simulink model "x2025_bolier_grupa_07"  (R2023b)
settings: Solver=VariableStepAuto  StartTime=0.0  StopTime=7000  RelTol=1e-3
model workspace (MAT data in the model file):
  Cd = 180
  Csh = 30
  K = 3.1616
  Tauf = 5
  Tf = 8
  Tfuel = 8
  Tw = 6
  k = 3.1616
values from neighbouring files (symbols this model uses):
  A1 = [-1/Tf 0 0 0 ... (first row only)    [Linearyzacja.m]
  A_prim = expm(A1*Ti)    [Dyskretyzacja.m]
  B1 = [1/Tf 0 ... (first row only)    [Linearyzacja.m]
  B_prim = integ*B1    [Dyskretyzacja.m]
  C1 = [0 0 CV 0 ... (first row only)    [Linearyzacja.m]
  CV = 0.5    [Linearyzacja.m]
  CV_FINAL_VALUE = 0.50    (= 0.5)    [INPUT.m]
  CV_INIT_VALUE = 0.5    [INPUT.m]
  D1 = [0 Pt_const ... (first row only)    [Linearyzacja.m]
  Pd_const = 1.025    [Linearyzacja.m]
  SIG = 0.5    [Linearyzacja.m]
  SIG_FINAL_VALUE = 0.3    [INPUT.m]
  SIG_INIT_VALUE = 0.5    [INPUT.m]
  STEP_TIME = 4000    [INPUT.m]
  Ti = 50.0    (= 50)    [Dyskretyzacja.m]
settings Model: Creator=jakub  LastModifiedBy=Filip

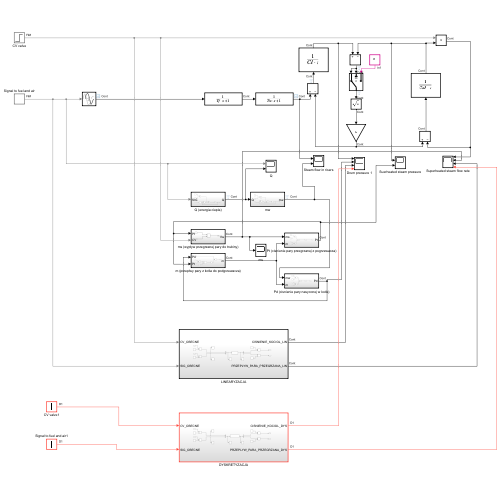
[thumbnail: Simulink's stored preview of the top-level diagram]
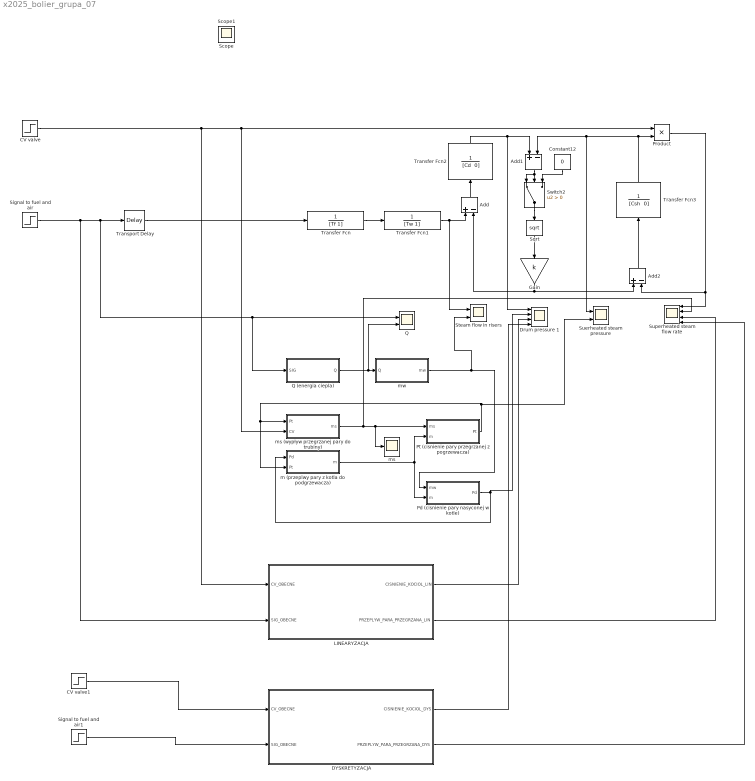
== system x2025_bolier_grupa_07 ==
  " mw " : Subsystem
  Add : Sum  Inputs=+-
  Add1 : Sum  Inputs=+-
  Add2 : Sum  Inputs=+-
  CV valve : Step  Time=STEP_TIME  Before=CV_INIT_VALUE  After=CV_FINAL_VALUE  SampleTime=0
  CV valve1 : Step  Time=STEP_TIME  Before=CV_INIT_VALUE  After=CV_FINAL_VALUE  SampleTime=Ti
  Constant12 : Constant  Value=0
  DYSKRETYZACJA : Subsystem
  Drum pressure 1 : Scope  NumInputPorts=4
  Gain : Gain  Gain=k
  LINEARYZACJA : Subsystem
  Pd (cisnienie pary nasyconej w kotle) : Subsystem
  Product : Product
  Pt (cisnienie pary przegrzanej z pogrzewacza) : Subsystem
  Q : Scope  NumInputPorts=2
  Q (energia ciepla) : Subsystem
  Signal to fuel and air : Step  Time=STEP_TIME  Before=SIG_INIT_VALUE  After=SIG_FINAL_VALUE  SampleTime=0
  Signal to fuel and air1 : Step  Time=STEP_TIME  Before=SIG_INIT_VALUE  After=SIG_FINAL_VALUE  SampleTime=Ti
  Sqrt : Sqrt
  Steam flow in risers : Scope  NumInputPorts=2
  Suerheated steam pressure : Scope  NumInputPorts=2
  Superheated steam flow rate : Scope  NumInputPorts=4
  Switch2 : Switch  Criteria=u2 > Threshold  SaturateOnIntegerOverflow=off  InputSameDT=off
  Transfer Fcn : TransferFcn  Denominator=[Tf 1]
  Transfer Fcn1 : TransferFcn  Denominator=[Tw 1]
  Transfer Fcn2 : TransferFcn  Denominator="[Cd  0]"
  Transfer Fcn3 : TransferFcn  Denominator="[Csh  0]"
  Transport Delay : TransportDelay  DelayTime=Tauf
  m (przeplwy pary z kotla do podgrzewacza) : Subsystem
  ms : Scope
  ms (wypływ przegrzanej pary do trubiny) : Subsystem
  Scope : Scope
  Scope1 : Scope
  wires:
  Transfer Fcn3/1 -> Suerheated steam pressure/1, Add1/2, Product/2
  Add2/1 -> Transfer Fcn3/1
  Product/1 -> Superheated steam flow rate/1, Add2/2
  Gain/1 -> Add2/1, Add/2
  CV valve/1 -> LINEARYZACJA/1(CV_OBECNE), Product/1, ms (wypływ przegrzanej pary do trubiny)/2(CV)
  Transport Delay/1 -> Transfer Fcn/1
  Signal to fuel and air/1 -> LINEARYZACJA/2(SIG_OBECNE), Transport Delay/1, Q/1, Q (energia ciepla)/1(SIG)
  Transfer Fcn2/1 -> Drum pressure 1/1, Add1/1
  Transfer Fcn1/1 -> Steam flow in risers/1, Add/1
  Add/1 -> Transfer Fcn2/1
  Sqrt/1 -> Gain/1
  Transfer Fcn/1 -> Transfer Fcn1/1
  Q (energia ciepla)/1(Q) -> Q/2, " mw "/1(Q)
  ms (wypływ przegrzanej pary do trubiny)/1(ms) -> Superheated steam flow rate/2, ms/1, Pt (cisnienie pary przegrzanej z pogrzewacza)/1(ms)
  Pt (cisnienie pary przegrzanej z pogrzewacza)/1(Pt) -> Suerheated steam pressure/2, ms (wypływ przegrzanej pary do trubiny)/1(Pt), m (przeplwy pary z kotla do podgrzewacza)/2(Pt)
  m (przeplwy pary z kotla do podgrzewacza)/1(m) -> Pd (cisnienie pary nasyconej w kotle)/2(m), Pt (cisnienie pary przegrzanej z pogrzewacza)/2(m)
  " mw "/1(mw) -> Steam flow in risers/2, Pd (cisnienie pary nasyconej w kotle)/1(mw)
  Pd (cisnienie pary nasyconej w kotle)/1(Pd) -> m (przeplwy pary z kotla do podgrzewacza)/1(Pd), Drum pressure 1/2
  Add1/1 -> Switch2/1, Switch2/2
  Switch2/1 -> Sqrt/1
  Constant12/1 -> Switch2/3
  LINEARYZACJA/1(CISNIENIE_KOCIOL_LIN) -> Drum pressure 1/3
  LINEARYZACJA/2(PRZEPLYW_PARA_PRZEGRZANA_LIN) -> Superheated steam flow rate/3
  CV valve1/1 -> DYSKRETYZACJA/1(CV_OBECNE)
  Signal to fuel and air1/1 -> DYSKRETYZACJA/2(SIG_OBECNE)
  DYSKRETYZACJA/1(CISNIENIE_KOCIOL_DYS) -> Drum pressure 1/4
  DYSKRETYZACJA/2(PRZEPLYW_PARA_PRZEGRZANA_DYS) -> Superheated steam flow rate/4

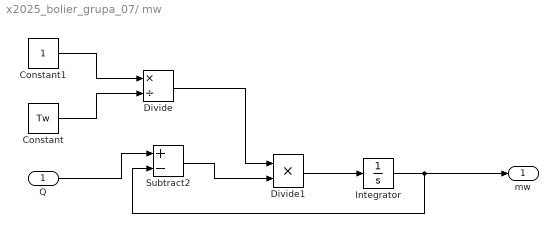
== system x2025_bolier_grupa_07/ mw  ==
  Q : Inport
  Constant : Constant  Value=Tw
  Constant1 : Constant
  Divide : Product  Inputs=*/
  Divide1 : Product  Inputs=**  RndMeth=Zero  SaturateOnIntegerOverflow=on
  Integrator : Integrator
  Subtract2 : Sum  Inputs=+-
  mw : Outport
  wires:
  Divide/1 -> Divide1/1
  Constant1/1 -> Divide/1
  Constant/1 -> Divide/2
  Divide1/1 -> Integrator/1
  Integrator/1 -> Subtract2/2, mw/1
  Q/1 -> Subtract2/1
  Subtract2/1 -> Divide1/2

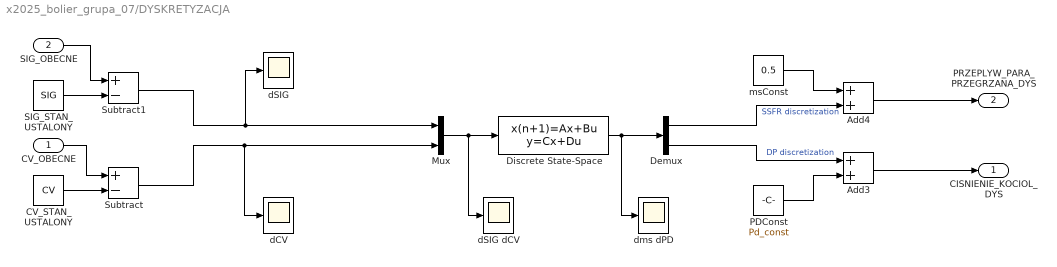
== system x2025_bolier_grupa_07/DYSKRETYZACJA ==
  CV_OBECNE : Inport
  SIG_OBECNE : Inport  Port=2
  Add3 : Sum
  Add4 : Sum
  CV_STAN_USTALONY : Constant  Value=CV
  Demux : Demux  Outputs=2
  Discrete State-Space : DiscreteStateSpace  A=A_prim  B=B_prim  C=C1  D=D1  SampleTime=-1
  Mux : Mux  Inputs=2
  PDConst : Constant  Value=Pd_const
  SIG_STAN_USTALONY : Constant  Value=SIG
  Subtract : Sum  Inputs=+-
  Subtract1 : Sum  Inputs=+-
  dCV : Scope
  dSIG : Scope
  dSIG dCV : Scope
  dms dPD : Scope
  msConst : Constant  Value=0.5
  CISNIENIE_KOCIOL_DYS : Outport
  PRZEPLYW_PARA_PRZEGRZANA_DYS : Outport  Port=2
  wires:
  Subtract1/1 -> dSIG/1, Mux/1
  Mux/1 -> Discrete State-Space/1, dSIG dCV/1
  CV_OBECNE/1 -> Subtract/1
  CV_STAN_USTALONY/1 -> Subtract/2
  PDConst/1 -> Add3/2
  Subtract/1 -> dCV/1, Mux/2
  Demux/2 -> Add3/1  "DP discretization"
  Discrete State-Space/1 -> dms dPD/1, Demux/1
  SIG_STAN_USTALONY/1 -> Subtract1/2
  Demux/1 -> Add4/2  "SSFR discretization"
  msConst/1 -> Add4/1
  Add3/1 -> CISNIENIE_KOCIOL_DYS/1
  SIG_OBECNE/1 -> Subtract1/1
  Add4/1 -> PRZEPLYW_PARA_PRZEGRZANA_DYS/1

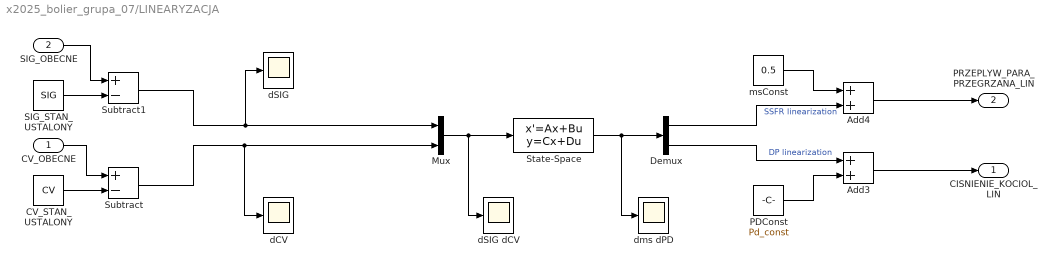
== system x2025_bolier_grupa_07/LINEARYZACJA ==
  CV_OBECNE : Inport
  SIG_OBECNE : Inport  Port=2
  Add3 : Sum
  Add4 : Sum
  CV_STAN_USTALONY : Constant  Value=CV
  Demux : Demux  Outputs=2
  Mux : Mux  Inputs=2
  PDConst : Constant  Value=Pd_const
  SIG_STAN_USTALONY : Constant  Value=SIG
  State-Space : StateSpace  A=A1  B=B1  C=C1  D=D1  InitialCondition=0  AllowTunableDMatrix=on
  Subtract : Sum  Inputs=+-
  Subtract1 : Sum  Inputs=+-
  dCV : Scope
  dSIG : Scope
  dSIG dCV : Scope
  dms dPD : Scope
  msConst : Constant  Value=0.5
  CISNIENIE_KOCIOL_LIN : Outport
  PRZEPLYW_PARA_PRZEGRZANA_LIN : Outport  Port=2
  wires:
  Subtract1/1 -> dSIG/1, Mux/1
  Mux/1 -> dSIG dCV/1, State-Space/1
  CV_OBECNE/1 -> Subtract/1
  CV_STAN_USTALONY/1 -> Subtract/2
  PDConst/1 -> Add3/2
  Subtract/1 -> dCV/1, Mux/2
  Demux/2 -> Add3/1  "DP linearization"
  State-Space/1 -> dms dPD/1, Demux/1
  SIG_STAN_USTALONY/1 -> Subtract1/2
  Demux/1 -> Add4/2  "SSFR linearization"
  msConst/1 -> Add4/1
  Add3/1 -> CISNIENIE_KOCIOL_LIN/1
  SIG_OBECNE/1 -> Subtract1/1
  Add4/1 -> PRZEPLYW_PARA_PRZEGRZANA_LIN/1

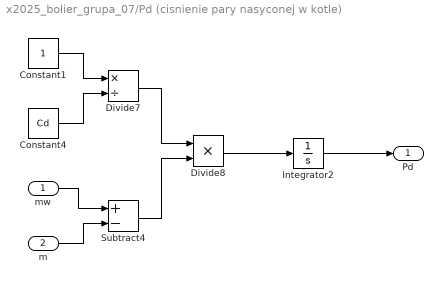
== system x2025_bolier_grupa_07/Pd (cisnienie pary nasyconej w kotle) ==
  mw : Inport
  m : Inport  Port=2
  Constant1 : Constant
  Constant4 : Constant  Value=Cd
  Divide7 : Product  Inputs=*/
  Divide8 : Product  Inputs=**
  Integrator2 : Integrator
  Subtract4 : Sum  Inputs=+-
  Pd : Outport
  wires:
  mw/1 -> Subtract4/1
  m/1 -> Subtract4/2
  Constant4/1 -> Divide7/2
  Constant1/1 -> Divide7/1
  Subtract4/1 -> Divide8/2
  Divide7/1 -> Divide8/1
  Divide8/1 -> Integrator2/1
  Integrator2/1 -> Pd/1

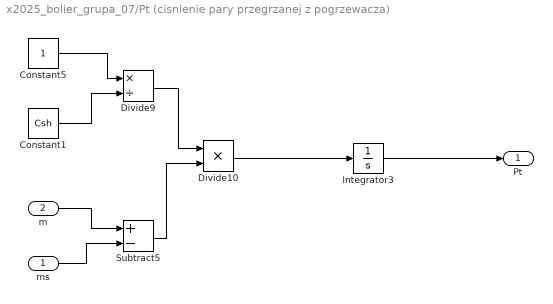
== system x2025_bolier_grupa_07/Pt (cisnienie pary przegrzanej z pogrzewacza) ==
  ms : Inport
  m : Inport  Port=2
  Constant1 : Constant  Value=Csh
  Constant5 : Constant
  Divide10 : Product  Inputs=**
  Divide9 : Product  Inputs=*/
  Integrator3 : Integrator
  Subtract5 : Sum  Inputs=+-
  Pt : Outport
  wires:
  ms/1 -> Subtract5/2
  m/1 -> Subtract5/1
  Constant1/1 -> Divide9/2
  Constant5/1 -> Divide9/1
  Divide9/1 -> Divide10/1
  Subtract5/1 -> Divide10/2
  Divide10/1 -> Integrator3/1
  Integrator3/1 -> Pt/1

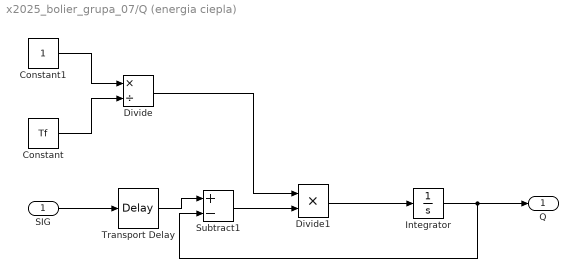
== system x2025_bolier_grupa_07/Q (energia ciepla) ==
  SIG : Inport
  Constant : Constant  Value=Tf
  Constant1 : Constant
  Divide : Product  Inputs=*/
  Divide1 : Product  Inputs=**  RndMeth=Zero  SaturateOnIntegerOverflow=on
  Integrator : Integrator
  Subtract1 : Sum  Inputs=+-
  Transport Delay : TransportDelay  DelayTime=Tauf
  Q : Outport
  wires:
  SIG/1 -> Transport Delay/1
  Transport Delay/1 -> Subtract1/1
  Subtract1/1 -> Divide1/2
  Constant1/1 -> Divide/1
  Constant/1 -> Divide/2
  Divide/1 -> Divide1/1
  Divide1/1 -> Integrator/1
  Integrator/1 -> Subtract1/2, Q/1

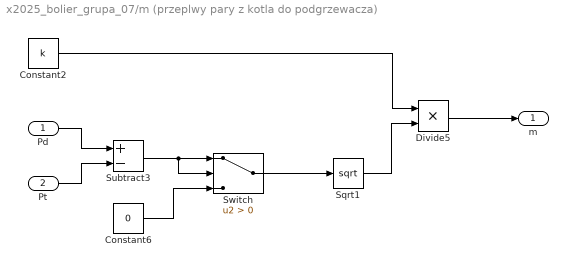
== system x2025_bolier_grupa_07/m (przeplwy pary z kotla do podgrzewacza) ==
  Pd : Inport
  Pt : Inport  Port=2
  Constant2 : Constant  Value=k
  Constant6 : Constant  Value=0
  Divide5 : Product  Inputs=**
  Sqrt1 : Sqrt
  Subtract3 : Sum  Inputs=+-
  Switch : Switch  Criteria=u2 > Threshold  SaturateOnIntegerOverflow=off  InputSameDT=off
  m : Outport
  wires:
  Pd/1 -> Subtract3/1
  Pt/1 -> Subtract3/2
  Constant6/1 -> Switch/3
  Subtract3/1 -> Switch/1, Switch/2
  Switch/1 -> Sqrt1/1
  Constant2/1 -> Divide5/1
  Sqrt1/1 -> Divide5/2
  Divide5/1 -> m/1

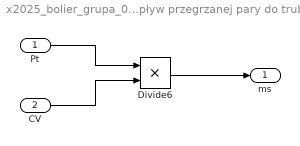
== system x2025_bolier_grupa_07/ms (wypływ przegrzanej pary do trubiny) ==
  Pt : Inport
  CV : Inport  Port=2
  Divide6 : Product  Inputs=**
  ms : Outport
  wires:
  Pt/1 -> Divide6/1
  CV/1 -> Divide6/2
  Divide6/1 -> ms/1
